simulink model "soc_range_doppler_fpga"  (R2025b)
settings: Solver=FixedStepDiscrete  StartTime=0.0  StopTime=inf  FixedStep=1/FPGAClkRate  RelTol=1e-3
values from neighbouring files (symbols this model uses):
  FPGAClkRate = Fs / SamplesPerClockCycle    (= 125000000)    [fmcw_run_test.m]    (also in soc_fmcw_init.m = 200000000)
  pulsePeriodSamples = ChirpSamples + 50    (= 1074)    [soc_range_doppler_system_param_init.m]    (also in soc_range_doppler_system_param_init_PDR_backup.m = 1952)
  pulseWidthSamples = 32    [soc_range_doppler_system_param_init.m]    (also in soc_range_doppler_system_param_init_PDR_backup.m)
  RngDimLen = ChirpSamples    (= 1024)    [soc_fmcw_init.m]    (also in soc_range_doppler_system_param_init.m; soc_range_doppler_system_param_init_PDR_backup.m)
  RxActiveSamples = ChirpSamples    (= 1024)    [soc_range_doppler_system_param_init.m]    (also in soc_range_doppler_system_param_init_PDR_backup.m)
  SamplesPerClockCycle = 2    [fmcw_run_test.m]    (also in soc_fmcw_init.m)
  TsFPGA = 1 / FPGAClkRate    (= 5e-09)    [soc_fmcw_init.m]
  txSignal = exp(1j * chirpPhase_short)    [soc_range_doppler_system_param_init.m]    (also in soc_range_doppler_system_param_init_PDR_backup.m = txSignalFullPeriod(1:pulseWidthSamples))
  VelDimLen = CPILength    (= 256)    [soc_fmcw_init.m]    (also in soc_range_doppler_system_param_init.m = 64; soc_range_doppler_system_param_init_PDR_backup.m = 64)
undefined symbols (not defined in the file or in its folder): NumBits1, NumBits2, TargetEmulator_MaxDelayLength, TargetEmulator_NCO_out_wl, TargetEmulator_NumChannels
libraries: simulink x9, socmemlib x8, hdlsllib x7, hwlogicconnlib x3, dsphdlsigops2 x1
(part 2 of 2)

== system soc_range_doppler_fpga/Radar Target Emulator/Multiple Target Emulator/Variable Delay RAM-based/Variable Delay RAM Based/RAM_ctrl ==
  idx : Inport
  valid_in : Inport  Port=2
  rd_addr_ctrl : Subsystem
  wr_addr_ctrl : Subsystem
  wr_addr : Outport  VectorParamsAs1DForOutWhenUnconnected=off
  wr_en : Outport  Port=2  VectorParamsAs1DForOutWhenUnconnected=off
  rd_addr : Outport  Port=3  VectorParamsAs1DForOutWhenUnconnected=off
  wires:
  idx/1 -> rd_addr_ctrl/2(idx)
  rd_addr_ctrl/1(rd_addr) -> rd_addr/1
  wr_addr_ctrl/1(wr_addr) -> wr_addr/1, rd_addr_ctrl/1(wr_addr)
  valid_in/1 -> wr_en/1, wr_addr_ctrl/1(valid_in)

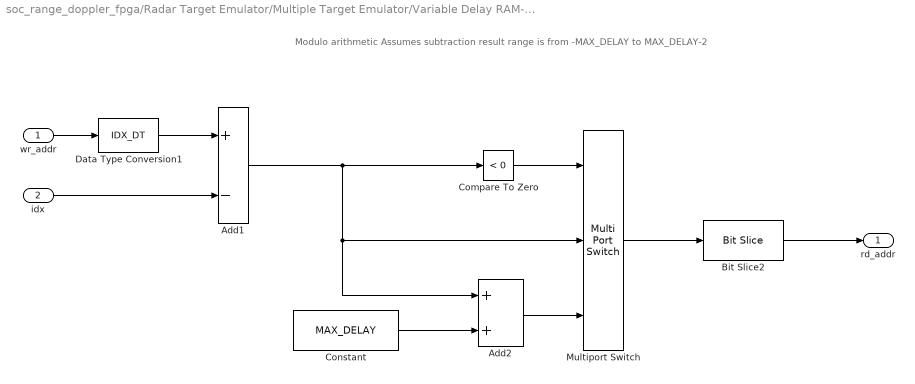
== system soc_range_doppler_fpga/Radar Target Emulator/Multiple Target Emulator/Variable Delay RAM-based/Variable Delay RAM Based/RAM_ctrl/rd_addr_ctrl ==
  note: Modulo arithmetic
      | Assumes subtraction result range is from -MAX_DELAY to MAX_DELAY-2
  wr_addr : Inport
  idx : Inport  Port=2
  Add1 : Sum  Inputs=+-
  Add2 : Sum
  Bit Slice2 : hdlsllib/Logic and Bit Operations/Bit Slice  lidx=ADDR_WIDTH-1  ridx=0
  Compare To Zero : simulink/Logic and Bit Operations/Compare To Zero  relop=<  OutDataTypeStr=boolean
  Constant : Constant  Value=MAX_DELAY  OutDataTypeStr=IDX_DT  SampleTime=-1
  Data Type Conversion1 : DataTypeConversion  OutDataTypeStr=IDX_DT  SaturateOnIntegerOverflow=off  RndMeth=Floor
  Multiport Switch : MultiPortSwitch  DataPortOrder=Zero-based contiguous  Inputs=2  zeroidx=on  SaturateOnIntegerOverflow=off  InputSameDT=off
  rd_addr : Outport  VectorParamsAs1DForOutWhenUnconnected=off
  wires:
  idx/1 -> Add1/2
  wr_addr/1 -> Data Type Conversion1/1
  Data Type Conversion1/1 -> Add1/1
  Add1/1 -> Add2/1, Multiport Switch/2, Compare To Zero/1
  Compare To Zero/1 -> Multiport Switch/1
  Constant/1 -> Add2/2
  Add2/1 -> Multiport Switch/3
  Multiport Switch/1 -> Bit Slice2/1
  Bit Slice2/1 -> rd_addr/1

== system soc_range_doppler_fpga/Radar Target Emulator/Multiple Target Emulator/Variable Delay RAM-based/Variable Delay RAM Based/RAM_ctrl/wr_addr_ctrl ==
  valid_in : Inport
  Constant : Constant  Value=MAX_DELAY-1  OutDataTypeStr=ADDR_DT  SampleTime=-1
  HDL Counter : hdlsllib/Sources/HDL Counter  CountType=Free running  CountInit=0  CountStep=1  CountMax=25  CountFromType=Initial value  CountFrom=0  CountResetPort=on  CountLoadPort=off  CountEnbPort=on  CountDirPort=off  CountHitOutputPort=off  CountDataType=Unsigned  CountWordLen=ADDR_WIDTH  CountFracLen=0  CountSampTime=1
  Logical Operator : Logic  IconShape=distinctive  AllPortsSameDT=off  OutDataTypeStr=boolean
  Relational Operator : RelationalOperator  Operator===  OutDataTypeStr=boolean  RndMeth=Simplest  InputSameDT=off
  wr_addr : Outport  VectorParamsAs1DForOutWhenUnconnected=off
  wires:
  Relational Operator/1 -> Logical Operator/1
  Logical Operator/1 -> HDL Counter/1
  Constant/1 -> Relational Operator/1
  valid_in/1 -> HDL Counter/2, Logical Operator/2
  HDL Counter/1 -> wr_addr/1, Relational Operator/2

== matlab function soc_range_doppler_fpga/Radar Target Emulator/Multiple Target Emulator/Variable Delay RAM-based/Variable Delay RAM Based/Set Complexity ==
  settings: fimath=hdlfimath
  data: ref input; din input; dout output
function dout = fcn(ref,din)
%#codegen

dout = cast(din,'like',ref);

== matlab function soc_range_doppler_fpga/Range Doppler Tx-Rx/ADC Interface/Unpack Vector I/MATLAB Function ==
  data: packed_in input; vec_out output; OutputWordLength parameter; VectorLength parameter
function vec_out = unpack_vector(packed_in, OutputWordLength, VectorLength)
%#codegen

OUT_WL = coder.const(OutputWordLength);
NUM_WORDS = coder.const(VectorLength);

packed_in_fi = cast_to_fi(packed_in);

temp = coder.nullcopy(fi(zeros(NUM_WORDS,1), 0,OUT_WL,0));
coder.unroll();
for ii=1:NUM_WORDS
   temp(ii) = bitsliceget(packed_in_fi, (ii-1)*OUT_WL + OUT_WL, (ii-1)*OUT_WL + 1);
end

vec_out = temp;

== matlab function soc_range_doppler_fpga/Range Doppler Tx-Rx/System Controller/System Controller Fcn ==
  data: cpi_start input; tx_active output; cpi_length input; rx_active output; rx_delay_cycles input; SamplesPerClockCycle parameter; RxActiveSamples parameter; pulseWidthSamples parameter; pulsePeriodSamples parameter
function [tx_active,rx_active] = ...
    sys_ctrl(cpi_start, cpi_length, rx_delay_cycles, ...
        SamplesPerClockCycle, RxActiveSamples, pulseWidthSamples, pulsePeriodSamples)

%% Constants
STATE_IDLE      = coder.const(fi(0, 0,2,0));
STATE_ACTIVE    = coder.const(fi(1, 0,2,0));
STATE_DONE      = coder.const(fi(2, 0,2,0));

RX_ACTIVE_CYCLES = coder.const(RxActiveSamples/SamplesPerClockCycle);
PULSE_PERIOD_CYCLES = coder.const(pulsePeriodSamples/SamplesPerClockCycle - 1);
PULSE_WIDTH_CYCLES = coder.const(pulseWidthSamples/SamplesPerClockCycle);

%% Initialize registers

persistent count_reg pulse_count_reg rx_active_end_reg
if isempty(count_reg)
    count_reg = fi(0, numerictype(0,nextpow2(PULSE_PERIOD_CYCLES),0), hdlfimath);
    pulse_count_reg = fi(0, numerictype(0,32,0), hdlfimath);
    rx_active_end_reg = fi(0, numerictype(0,32,0), hdlfimath);
end

persistent state_next
if isempty(state_next)
    state_next = STATE_IDLE;
end

%% Signals from registers
state = state_next;
count = count_reg;                  % count samples in a pulse period
pulse_count = pulse_count_reg;      % count number of pulse periods completed
rx_active_end = rx_active_end_reg;  % count value where rx active window ends

%% State machine logic

% Output defaults
tx_active = false;
rx_active = false;

switch state
    
    case STATE_IDLE
        if cpi_start
            state_next = STATE_ACTIVE;
            count_reg(:) = 0;
            pulse_count_reg(:) = 0;
            rx_active_end_reg(:) = rx_delay_cycles + RX_ACTIVE_CYCLES;
        end
        
    case STATE_ACTIVE
        if (count == PULSE_PERIOD_CYCLES)
            count_reg(:) = 0;
            if pulse_count == cpi_length
                state_next = STATE_DONE; 
            else
                pulse_count_reg(:) = pulse_count + 1;
            end
        else
            count_reg(:) = count + 1;
        end
        
        % Outputs
        if (count < PULSE_WIDTH_CYCLES)
            tx_active = true;
        end
        if (count >= rx_delay_cycles) && (count < rx_active_end)
            rx_active = true; 
        end
        
    case STATE_DONE
        if ~cpi_start
            state_next = STATE_IDLE;
        end
end

== matlab function soc_range_doppler_fpga/Range Doppler Tx-Rx/DAC Interface/Pack Vector Q/pack_vector ==
  data: u input; y output
function y = pack_vector(u)
%#codegen

assert(isreal(u),'Expected input to be real');

N = coder.const(numel(u));

temp = coder.nullcopy((cast_to_fi(zeros([N 1],'like',u))));

% Interleave real/imag
coder.unroll();
for ii=N:-1:1
    temp(N-ii+1) = u(ii);
end

y = bitconcat(temp);

== matlab function soc_range_doppler_fpga/Range Doppler Tx-Rx/DAC Interface/Pack Vector I/pack_vector ==
  data: u input; y output
function y = pack_vector(u)
%#codegen

assert(isreal(u),'Expected input to be real');

N = coder.const(numel(u));

temp = coder.nullcopy((cast_to_fi(zeros([N 1],'like',u))));

% Interleave real/imag
coder.unroll();
for ii=N:-1:1
    temp(N-ii+1) = u(ii);
end

y = bitconcat(temp);

== matlab function soc_range_doppler_fpga/Range Doppler Tx-Rx/DMA Interface/Pack Complex Vector/pack_vector_complex ==
  data: u input; y output
function y = pack_vector_complex(u)
%#codegen

assert(~isreal(u),'Expected input to be complex');

N = coder.const(numel(u));

temp = coder.nullcopy((cast_to_fi(zeros([N*2 1],'like',real(u)))));

% Interleave real/imag
coder.unroll();
for ii=N:-1:1
    temp((ii-1)*2+2) = real(u(N-ii+1));
    temp((ii-1)*2+1) = imag(u(N-ii+1));
end

y = bitconcat(temp);

== matlab function soc_range_doppler_fpga/Range Doppler Tx-Rx/ADC Interface/Unpack Vector Q/MATLAB Function ==
  data: packed_in input; vec_out output; OutputWordLength parameter; VectorLength parameter
function vec_out = unpack_vector(packed_in, OutputWordLength, VectorLength)
%#codegen

OUT_WL = coder.const(OutputWordLength);
NUM_WORDS = coder.const(VectorLength);

packed_in_fi = cast_to_fi(packed_in);

temp = coder.nullcopy(fi(zeros(NUM_WORDS,1), 0,OUT_WL,0));
coder.unroll();
for ii=1:NUM_WORDS
   temp(ii) = bitsliceget(packed_in_fi, (ii-1)*OUT_WL + OUT_WL, (ii-1)*OUT_WL + 1);
end

vec_out = temp;

== matlab function soc_range_doppler_fpga/Radar Target Emulator/Pack Data/Pack Vector/pack_vector ==
  data: u input; y output
function y = pack_vector(u)
%#codegen

assert(isreal(u),'Expected input to be real');

N = coder.const(numel(u));

temp = coder.nullcopy((cast_to_fi(zeros([N 1],'like',u))));

% Interleave real/imag
coder.unroll();
for ii=N:-1:1
    temp(N-ii+1) = u(ii);
end

y = bitconcat(temp);

== matlab function soc_range_doppler_fpga/Radar Target Emulator/Pack Data/Pack Vector1/pack_vector ==
  data: u input; y output
function y = pack_vector(u)
%#codegen

assert(isreal(u),'Expected input to be real');

N = coder.const(numel(u));

temp = coder.nullcopy((cast_to_fi(zeros([N 1],'like',u))));

% Interleave real/imag
coder.unroll();
for ii=N:-1:1
    temp(N-ii+1) = u(ii);
end

y = bitconcat(temp);

== matlab function soc_range_doppler_fpga/Radar Target Emulator/Multiple Target Emulator/Unpack Data/Unpack Vector/MATLAB Function ==
  data: packed_in input; vec_out output; OutputWordLength parameter; VectorLength parameter
function vec_out = unpack_vector(packed_in, OutputWordLength, VectorLength)
%#codegen

OUT_WL = coder.const(OutputWordLength);
NUM_WORDS = coder.const(VectorLength);

packed_in_fi = cast_to_fi(packed_in);

temp = coder.nullcopy(fi(zeros(NUM_WORDS,1), 0,OUT_WL,0));
coder.unroll();
for ii=1:NUM_WORDS
   temp(ii) = bitsliceget(packed_in_fi, (ii-1)*OUT_WL + OUT_WL, (ii-1)*OUT_WL + 1);
end

vec_out = temp;

== matlab function soc_range_doppler_fpga/Radar Target Emulator/Multiple Target Emulator/Unpack Data/Unpack Vector1/MATLAB Function ==
  data: packed_in input; vec_out output; OutputWordLength parameter; VectorLength parameter
function vec_out = unpack_vector(packed_in, OutputWordLength, VectorLength)
%#codegen

OUT_WL = coder.const(OutputWordLength);
NUM_WORDS = coder.const(VectorLength);

packed_in_fi = cast_to_fi(packed_in);

temp = coder.nullcopy(fi(zeros(NUM_WORDS,1), 0,OUT_WL,0));
coder.unroll();
for ii=1:NUM_WORDS
   temp(ii) = bitsliceget(packed_in_fi, (ii-1)*OUT_WL + OUT_WL, (ii-1)*OUT_WL + 1);
end

vec_out = temp;
